simulink model "trucksim_different_condition"  (R2023b)
settings: Solver=FixedStepAuto  StartTime=0.0  StopTime=5  FixedStep=0.001  RelTol=1e-3  EnableMultiTasking=on
InitFcn:
  | py.sys.path().insert(int32(0), 'D:\YRJ_Workspace\DDK-Trucksim-python\MPC');
libraries: Solver_SF x1
settings Model: Creator=dzY  LastModifiedBy=Admin
settings DataIOCC: SaveFormat=Array  ReturnWorkspaceOutputs=off
settings OptimizationCC: LifeSpan=inf
settings DebuggingCC: SolverPrmCheckMsg=warning  UnconnectedInputMsg=warning  UnconnectedOutputMsg=warning  UnconnectedLineMsg=warning  SFUnexpectedBacktrackingDiag=warning  SFNoUnconditionalDefaultTransitionDiag=warning  SFExecutionAtInitializationDiag=none  ArithmeticOperatorsInVariantConditions=warning
settings HardwareCC: ProdBitPerPointer=32  ProdBitPerSizeT=32  ProdBitPerPtrDiffT=32  ProdLargestAtomicFloat=None  ProdIntDivRoundTo=Undefined  ProdEndianess=Unspecified  ProdWordSize=32  ProdHWDeviceType=32-bit Generic
settings ModelReferenceCC: EnableRefExpFcnMdlSchedulingChecks=on  PropagateSignalLabelsOutOfModel=off
settings SFSimCC: SimUseLocalCustomCode=off  CustomCodeUndefinedFunction=UseInterfaceOnly
settings RTWCC: RTWUseLocalCustomCode=off
settings CodeAppCC: StateflowObjectComments=on
settings GRTTargetCC: TargetLangStandard=C89/C90 (ANSI)
settings ConfigComp: CovMetricSettings=dw  CovSaveCumulativeToWorkspaceVar=on  CovSaveSingleToWorkspaceVar=on  CovExternalEMLEnable=off  CovSFcnEnable=off

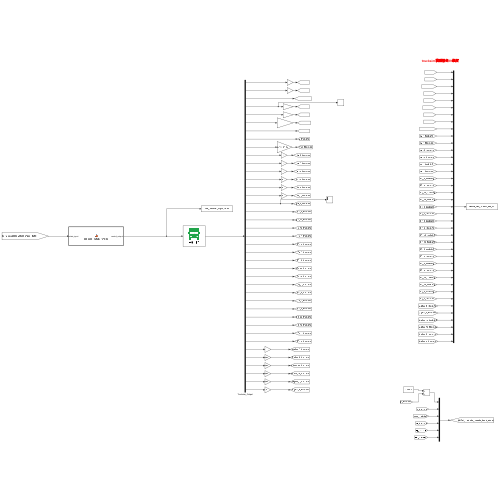
[thumbnail: Simulink's stored preview of the top-level diagram]
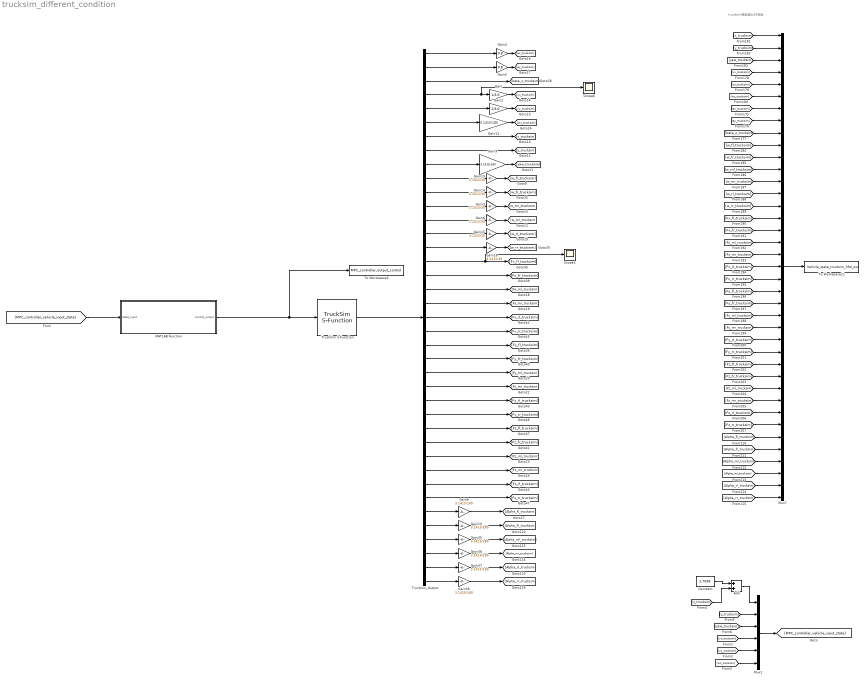
== system trucksim_different_condition ==
  note: trucksim模型输出39维度
  Add : Sum
  Constant : Constant  Value=2.7658
  Gain : Gain  Gain=1/3.6
  Gain{8..10,12,35..38} (8 alike) : Gain  Gain=3.1415/180
  Gain{3,6,13..16} (6 alike) : Gain  Gain=3.1415/30
  Gain2 : Gain  Gain=1/3.6
  Gain4 : Gain  Gain=9.8
  Gain5 : Gain  Gain=9.8
  MATLAB Function : MATLAB Function  TreatAsAtomicUnit=on
  Mux1 : Mux  Inputs=6
  Mux7 : Mux  Inputs=39
  Scope2 : Scope
  Scope6 : Scope
  To Workspace11 : ToWorkspace  VariableName=Vehicle_state_trucksim_39d_out  SaveFormat=Timeseries  SampleTime=-1
  To Workspace3 : ToWorkspace  VariableName=MPC_controller_output_control  SaveFormat=Timeseries  SampleTime=-1
  TruckSim S-Function : Solver_SF/TruckSim S-Function  Priority=1  SIMFILE=simfile.sim
      settings: SourceProductName=TruckSim S-Function
  Trucksim_Output : Demux  Outputs=39
  wires:
  Gain2/1 -> [vy_trucksim]
  Gain/1 -> [vx_trucksim]
  Gain9/1 -> [yaw_trucksim]
  Gain12/1 -> [wz_trucksim]
  Gain13/1 -> [w_fl_trucksim]
  Gain14/1 -> [w_fr_trucksim]
  Gain15/1 -> [w_rl_trucksim]
  Gain16/1 -> [w_rr_trucksim]
  Gain4/1 -> [ax_trucksim]
  Gain5/1 -> [ay_trucksim]
  Gain3/1 -> [w_ml_trucksim]
  Gain6/1 -> [w_mr_trucksim]
  Trucksim_Output/1 -> Gain4/1
  Trucksim_Output/2 -> Gain5/1
  Trucksim_Output/3 -> [beta_z_trucksim]
  Trucksim_Output/4 -> Scope6/1, Gain/1
  Trucksim_Output/5 -> Gain2/1
  Trucksim_Output/6 -> Gain12/1
  Trucksim_Output/7 -> [x_trucksim]
  Trucksim_Output/8 -> [y_trucksim]
  Trucksim_Output/9 -> Gain9/1
  Trucksim_Output/10 -> Gain13/1
  Trucksim_Output/11 -> Gain14/1
  Trucksim_Output/12 -> Gain3/1
  Trucksim_Output/13 -> Gain6/1
  Trucksim_Output/14 -> Gain15/1
  Trucksim_Output/15 -> Gain16/1
  Trucksim_Output/16 -> Scope2/1, [Fx_fl_trucksim]
  Trucksim_Output/17 -> [Fx_fr_trucksim]
  Trucksim_Output/18 -> [Fx_ml_trucksim]
  Trucksim_Output/19 -> [Fx_mr_trucksim]
  Trucksim_Output/20 -> [Fx_rl_trucksim]
  Trucksim_Output/21 -> [Fx_rr_trucksim]
  Trucksim_Output/22 -> [Fy_fl_trucksim]
  Trucksim_Output/23 -> [Fy_fr_trucksim]
  Trucksim_Output/24 -> [Fy_ml_trucksim]
  Trucksim_Output/25 -> [Fy_mr_trucksim]
  Trucksim_Output/26 -> [Fy_rl_trucksim]
  Trucksim_Output/27 -> [Fy_rr_trucksim]
  Trucksim_Output/28 -> [Fz_fl_trucksim]
  Trucksim_Output/29 -> [Fz_fr_trucksim]
  Trucksim_Output/30 -> [Fz_ml_trucksim]
  Trucksim_Output/31 -> [Fz_mr_trucksim]
  Trucksim_Output/32 -> [Fz_rl_trucksim]
  Trucksim_Output/33 -> [Fz_rr_trucksim]
  [x_trucksim] -> Mux7/1
  [y_trucksim] -> Mux7/2
  [yaw_trucksim] -> Mux7/3
  [vx_trucksim] -> Mux7/4
  [vy_trucksim] -> Mux7/5
  [wz_trucksim] -> Mux7/6
  [ax_trucksim] -> Mux7/7
  [ay_trucksim] -> Mux7/8
  [beta_z_trucksim] -> Mux7/9
  [w_fl_trucksim] -> Mux7/10
  [w_fr_trucksim] -> Mux7/11
  [w_ml_trucksim] -> Mux7/12
  [w_mr_trucksim] -> Mux7/13
  [w_rl_trucksim] -> Mux7/14
  [w_rr_trucksim] -> Mux7/15
  [Fx_fl_trucksim] -> Mux7/16
  [Fx_fr_trucksim] -> Mux7/17
  [Fx_ml_trucksim] -> Mux7/18
  [Fx_mr_trucksim] -> Mux7/19
  [Fx_rl_trucksim] -> Mux7/20
  [Fx_rr_trucksim] -> Mux7/21
  [Fy_fl_trucksim] -> Mux7/22
  [Fy_fr_trucksim] -> Mux7/23
  [Fy_ml_trucksim] -> Mux7/24
  [Fy_mr_trucksim] -> Mux7/25
  [Fy_rl_trucksim] -> Mux7/26
  [Fy_rr_trucksim] -> Mux7/27
  [Fz_fl_trucksim] -> Mux7/28
  [Fz_fr_trucksim] -> Mux7/29
  [Fz_ml_trucksim] -> Mux7/30
  [Fz_mr_trucksim] -> Mux7/31
  [Fz_rl_trucksim] -> Mux7/32
  [Fz_rr_trucksim] -> Mux7/33
  Mux7/1 -> To Workspace11/1
  TruckSim S-Function/1 -> Trucksim_Output/1
  [Alpha_fl_trucksim] -> Mux7/34
  [Alpha_fr_trucksim] -> Mux7/35
  [Alpha_ml_trucksim] -> Mux7/36
  [Alpha_mr_trucksim] -> Mux7/37
  [Alpha_rl_trucksim] -> Mux7/38
  [Alpha_rr_trucksim] -> Mux7/39
  Trucksim_Output/34 -> Gain8/1
  Gain8/1 -> [Alpha_fl_trucksim]
  Trucksim_Output/35 -> Gain10/1
  Gain10/1 -> [Alpha_fr_trucksim]
  Trucksim_Output/36 -> Gain35/1
  Gain35/1 -> [Alpha_ml_trucksim]
  Trucksim_Output/37 -> Gain36/1
  Gain36/1 -> [Alpha_mr_trucksim]
  Trucksim_Output/38 -> Gain37/1
  Gain37/1 -> [Alpha_rl_trucksim]
  Trucksim_Output/39 -> Gain38/1
  Gain38/1 -> [Alpha_rr_trucksim]
  MATLAB Function/1(control_output) -> To Workspace3/1, TruckSim S-Function/1
  [y_trucksim] -> Mux1/2
  [yaw_trucksim] -> Mux1/3
  [vx_trucksim] -> Mux1/4
  [vy_trucksim] -> Mux1/5
  [wz_trucksim] -> Mux1/6
  Mux1/1 -> [MPC_controller_vehicle_input_state]
  [MPC_controller_vehicle_input_state] -> MATLAB Function/1(state_input)
  [x_trucksim] -> Add/2
  Constant/1 -> Add/1
  Add/1 -> Mux1/1

== matlab function trucksim_different_condition/MATLAB Function ==
  data: state_input input; control_output output
% MATLAB Function模块包装器
% 用于在Simulink中调用Python MPC控制器（Koopman-MPC V2：新网络 + 新MPC）
%
% 使用方法：
% 1. 在Simulink中添加"MATLAB Function"块
% 2. 将此代码复制到MATLAB Function块中
% 3. 配置输入输出端口
% 4. 在Model Callbacks的InitFcn中添加Python路径：
%    py.sys.path().insert(int32(0), 'D:\YRJ_Workspace\DDK-Trucksim-python\MPC');

function control_output = ddk_mpc_matlab_function(state_input)
%#codegen
% Koopman-MPC V2 控制器 MATLAB Function 包装器（Trucksim）
% 新 ckpt：CustomEncoderUnscaledv2WithoutNorm + KoopmanMPC（12维控制、硬约束）
%
% 输入:
%   state_input: [6x1] 车辆状态（相对起点）[X(m), Y(m), Yaw(rad), vx(m/s), vy(m/s), yaw_rate(rad/s)]
%
% 输出:
%   control_output: [12x1] [steer_LF..RR(deg), torque_LF..RR(N·m)]

% 显式声明输入输出大小（帮助代码生成器确定维度）
assert(isequal(size(state_input), [6, 1]), 'state_input must be 6x1');
control_output = zeros(12, 1);  % 预分配输出大小（Trucksim为12维）

% 声明Python函数为外部函数（不参与代码生成）
coder.extrinsic('py.ddk_mpc_sfunction.initialize_controller');
coder.extrinsic('py.ddk_mpc_sfunction.compute_control');
coder.extrinsic('py.ddk_mpc_sfunction.reset_controller');

% 持久变量（在仿真过程中保持状态）
persistent is_initialized;
persistent param_path;
persistent data_path;

% 初始化（第一次调用时）
% 注意：Python路径配置必须在Simulink运行前在MATLAB命令窗口执行：
% py.sys.path().insert(int32(0), 'D:\YRJ_Workspace\DDK-Trucksim-python\MPC');
% 或者在Model Callbacks的InitFcn中添加上述命令
if isempty(is_initialized)
    is_initialized = false;
    
    % 新 ckpt 路径（与 mpc_dk 一致，项目根下 ckpt 文件夹）
    param_path = 'D:\YRJ_Workspace\DDK-Trucksim-python\ckpt\DeepEDMD-Transv2wonorm-hd16-multiset-100e-remote-local-lr1e-4-rollover-0.05pilossv24-0222.pth';
    
    % 参考轨迹 .mat（支持 ref_trajectory / position+velocity / Pos+X 格式）
    data_path = 'D:\YRJ_Workspace\DDK-Trucksim-python\data\ref_traj\all\all_wheel_steer_Scenario_snake_acc_5m_s_ref.mat';
    
    % ---------- Q / R / I 超参数（可选，传入 Python 用于 MPC 代价权重）----------
    % Q: 状态/跟踪权重 [16]，前 6 维为物理状态 (x,y,yaw,vx,vy,wz)，后 10 维为 Koopman 提升维
    Q = [ones(6,1); ones(10,1)];   % 默认全 1；可改为标量或逐维
    % R: 控制偏离中性(0.5)的惩罚 [12]，前 6 转矩、后 6 转向
    R = 0.01 * ones(12, 1);        % 默认 0.01；增大可更保守
    % I: 控制增量/平滑惩罚 [12]
    I = 1.5 * ones(12, 1);         % 默认 0.5；增大可减轻抖动
    % 若希望使用 Python 端默认值，可将 Q、R、I 任一设为 []，例如: Q=[]; R=[]; I=[];
    
    % 初始化 Koopman-MPC V2：param_path, data_path, Np, Nc, sample_interval, decimation, Q, R, I
    % sample_interval=1 与 Koopman 0.01s 对齐；decimation=10 表示每 10 次调用求解一次 MPC
    py.ddk_mpc_sfunction.initialize_controller(param_path, data_path, 30, 30, 1, 10, Q, R, I);
    % 为避免Python侧全局状态在多次仿真间残留，初始化后显式重置一次状态
    % 重要：Python侧u_prev为“归一化控制”，应以0.5作为零转矩/零转角的初始值
    py.ddk_mpc_sfunction.reset_controller();
    is_initialized = true;
end

% 调用Python MPC控制器
% compute_control返回12维控制输出：
% [steer_LF(deg), steer_RF(deg), steer_LM(deg), steer_RM(deg), 
%  steer_LR(deg), steer_RR(deg),
%  torque_LF(N·m), torque_RF(N·m), torque_LM(N·m), torque_RM(N·m),
%  torque_LR(N·m), torque_RR(N·m)]
control_py = py.ddk_mpc_sfunction.compute_control(state_input);
control_output = double(control_py);
control_output = reshape(control_output(:), 12, 1);  % 确保输出为12x1

% 安全检查：确保输出维度正确
if numel(control_output) ~= 12
    warning('Control output dimension error, returning zero control');
    control_output = zeros(12, 1);
end

% 可选：添加控制输出限幅（如果需要）
% 转向角限制：±30度
control_output(1:6) = max(-30, min(30, control_output(1:6)));
% 转矩限制：根据实际车辆参数设置
control_output(7:12) = max(-1000, min(1000, control_output(7:12)));

end
